simulink model "tryout"  (R2021a)
settings: Solver=VariableStepAuto  StartTime=0.0  StopTime=10  RelTol=1e-3
values from neighbouring files (symbols this model uses):
  A = [0 0 1 0;0 0 0 1;1 0 0 -20;4.998 -70 -49.98 0]    [Controlib.m]    (also in Observ.m = [0 0 1 0; 0 0 0 1;1 0 0 -20;4.998 -70 -49.98 0]; Opp.m = double(subs(jac,[x1,x2,x3,x4],[op1,op2,op3,op4])); Stabili.m = [0 0 1 0; 0 0 0 1;1 0 0 -20;4.998 -70 -49.98 0]; lyaptesting.m = [0 0 1 0;0 0 0 1;1 0 0 -20;5 -70 -50 0])
  B = [0 0;0 0;F/7 0;0 M/2]    [Controlib.m]    (also in Linearization.m; Observ.m = [0 0;0 0 ;F/7 0 ; 0 M/2]; Opp.m; Stabili.m = [0 0;0 0; F/7 0; 0 M/2])
  C = [1 0 0 0 ;0 1 0 0]    [Controlib.m]    (also in Linearization.m = [1 0 0 0;0 1 0 0]; Observ.m = [1 0 0 0;0 1 0 0]; Opp.m = [1 0 0 0;0 1 0 0]; Stabili.m = [1 0 0 0; 0 1 0 0])
  K = place(A,B,PR)    [Poleplace.m]
  Ke = place(A',C',Pobs)'    [Stateobserv.m]
settings Model: Creator=bahet  LastModifiedBy=Musthafa

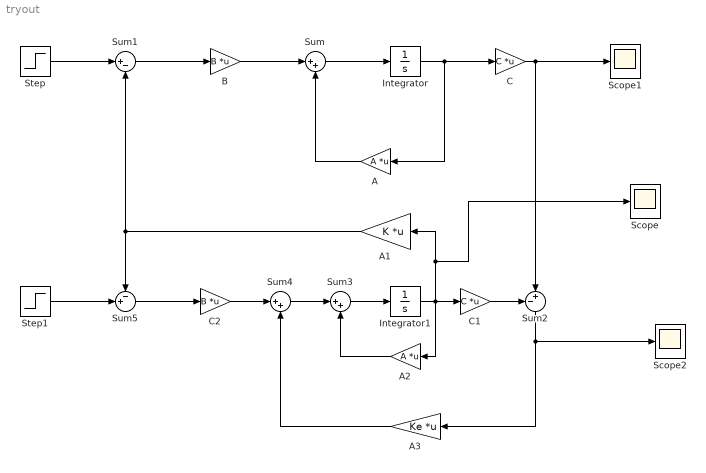
== system tryout ==
  A : Gain  Gain=A  Multiplication=Matrix(K*u)
  A1 : Gain  Gain=K  Multiplication=Matrix(K*u)
  A2 : Gain  Gain=A  Multiplication=Matrix(K*u)
  A3 : Gain  Gain=Ke  Multiplication=Matrix(K*u)
  B : Gain  Gain=B  Multiplication=Matrix(K*u)
  C : Gain  Gain=C  Multiplication=Matrix(K*u)
  C1 : Gain  Gain=C  Multiplication=Matrix(K*u)
  C2 : Gain  Gain=B  Multiplication=Matrix(K*u)
  Integrator : Integrator
  Integrator1 : Integrator
  Scope : Scope
  Scope1 : Scope
  Scope2 : Scope
  Step : Step  Time=0  After=[1;1]  SampleTime=0
  Step1 : Step  Time=0  After=[1;1]  SampleTime=0
  Sum : Sum  Inputs=|++
  Sum1 : Sum  Inputs=|+-
  Sum2 : Sum  Inputs=-+|
  Sum3 : Sum  Inputs=|++
  Sum4 : Sum  Inputs=|++
  Sum5 : Sum  Inputs=-+|
  wires:
  Integrator/1 -> C/1, A/1
  A/1 -> Sum/2
  Sum/1 -> Integrator/1
  B/1 -> Sum/1
  Sum1/1 -> B/1
  A1/1 -> Sum1/2, Sum5/1
  Step/1 -> Sum1/1
  Sum3/1 -> Integrator1/1
  C1/1 -> Sum2/1
  Sum4/1 -> Sum3/1
  C2/1 -> Sum4/1
  A2/1 -> Sum3/2
  A3/1 -> Sum4/2
  Sum2/1 -> A3/1, Scope2/1
  Sum5/1 -> C2/1
  Step1/1 -> Sum5/2
  C/1 -> Scope1/1, Sum2/2
  Integrator1/1 -> Scope/1, A1/1, C1/1, A2/1
